simulink model "plant_VV"  (R2023a)
settings: Solver=FixedStepAuto  StartTime=0.0  StopTime=10.0  FixedStep=0.01  RelTol=1e-3
values from neighbouring files (symbols this model uses):
  dt = 0.01    [untitled.m]
  sys = ss(A,B,C,D)    [control_law_design.m]    (also in untitled.m = ss(A,B,C,D, dt))
libraries: simulink_extras x4, shared6dof x1
settings Model: Creator=timme  LastModifiedBy=timme
settings OptimizationCC: BlockReduction=off  DefaultParameterBehavior=Inlined  BufferReuse=off

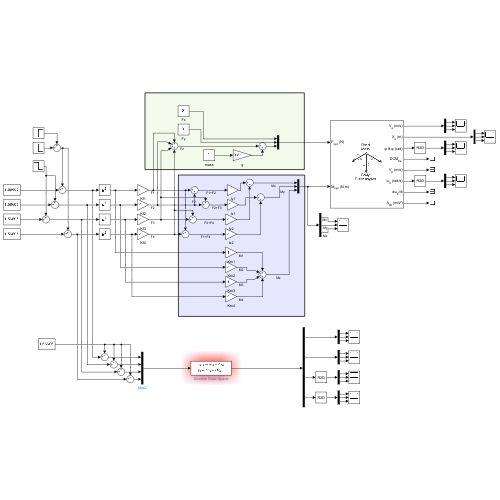
[thumbnail: Simulink's stored preview of the top-level diagram]
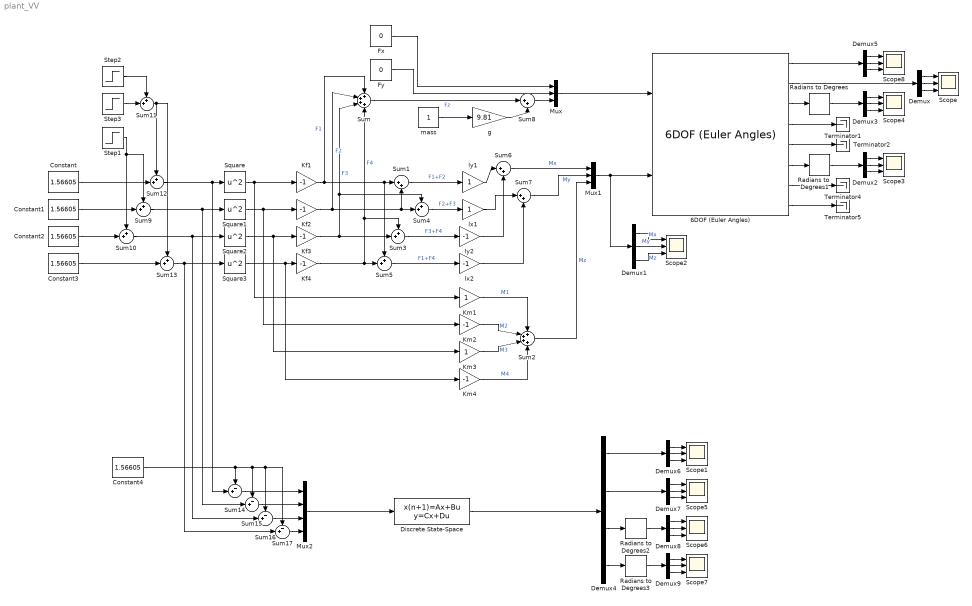
== system plant_VV ==
  6DOF (Euler Angles) : shared6dof/6DOF (Euler Angles)  units=Metric (MKS)  mtype=Fixed  rep=Euler Angles  xme_0=[0 0 0]  Vm_0=[0 0 0]  eul_0=[0 0 0]  pm_0=[0 0 0]  mass_0=1.0  mass_e=0.5  mass_f=2.0  inertia=eye(3)  inertia_e=eye(3)  inertia_f=2*eye(3)  k_quat=1.0  vre_flag=on  abi_flag=off  aMode=0  xme_statename=''  Vm_statename=''  eul_statename=''  quat_statename=''  pm_statename=''  mass_statename=''
  Constant{,1..4} (5 alike) : Constant  Value=1.56605
  Demux{,1..3,5..9} (9 alike) : Demux  Outputs=3
  Demux4 : Demux  Outputs=[3 3 3 3]
  Discrete State-Space : DiscreteStateSpace  A=sys.A  B=sys.B  C=sys.C  D=sys.D  SampleTime=dt
  Fx : Constant  Value=0
  Fy : Constant  Value=0
  Kf{1..4} (4 alike) : Gain  Gain=-1
  Km1 : Gain
  Km2 : Gain  Gain=-1
  Km3 : Gain
  Km4 : Gain  Gain=-1
  Mux : Mux  Inputs=3
  Mux1 : Mux  Inputs=3
  Mux2 : Mux
  Radians to Degrees{,1..3} (4 alike) : simulink_extras/Transformations/Radians to Degrees
  Scope{,1..8} (9 alike) : Scope  NumInputPorts=3
  Square{,1..3} (4 alike) : Math  Operator=square
  Step1 : Step  Time=0.05  Before=0.5  After=0  SampleTime=0
  Step2 : Step  Time=0.05  After=0.5  SampleTime=0
  Step3 : Step  Time=0.1  After=-0.5  SampleTime=0
  Sum : Sum  Inputs=++++
  Sum{1,6..8} (4 alike) : Sum  Inputs=|++
  Sum{3..5,9..13} (8 alike) : Sum  Inputs=++|
  Sum{14..17} (4 alike) : Sum  Inputs=-+|
  Sum2 : Sum  Inputs=++++
  Terminator{1..2,4..5} (4 alike) : Terminator
  g : Gain  Gain=9.81
  lx1 : Gain
  lx2 : Gain  Gain=-1
  ly1 : Gain
  ly2 : Gain  Gain=-1
  mass : Constant
  wires:
  6DOF (Euler Angles)/2 -> Demux/1
  Mux/1 -> 6DOF (Euler Angles)/1
  Constant/1 -> Sum12/2
  Constant1/1 -> Sum9/2
  Square/1 -> Kf1/1, Km1/1
  Square1/1 -> Km2/1, Kf2/1
  Constant2/1 -> Sum10/2
  Square2/1 -> Km3/1, Kf3/1
  Constant3/1 -> Sum13/2
  Square3/1 -> Km4/1, Kf4/1
  Sum/1 -> Sum8/1  "Fz"
  Fx/1 -> Mux/1
  Fy/1 -> Mux/2
  Kf1/1 -> Sum/1, Sum1/1, Sum5/1  "F1"
  Kf2/1 -> Sum/2, Sum4/2, Sum1/2  "F2"
  Kf4/1 -> Sum/4, Sum3/1, Sum5/2  "F4"
  Kf3/1 -> Sum/3, Sum4/1, Sum3/2  "F3"
  Mux1/1 -> Demux1/1, 6DOF (Euler Angles)/2
  Km1/1 -> Sum2/1  "M1"
  Km2/1 -> Sum2/2  "M2"
  Km3/1 -> Sum2/3  "M3"
  Km4/1 -> Sum2/4  "M4"
  Sum2/1 -> Mux1/3  "Mz"
  Sum5/1 -> lx2/1  "F1+F4"
  Sum3/1 -> ly2/1  "F3+F4"
  Sum4/1 -> lx1/1  "F2+F3"
  Sum1/1 -> ly1/1  "F1+F2"
  ly1/1 -> Sum6/1
  ly2/1 -> Sum6/2
  Sum6/1 -> Mux1/1  "Mx"
  Sum7/1 -> Mux1/2  "My"
  lx1/1 -> Sum7/1
  lx2/1 -> Sum7/2
  6DOF (Euler Angles)/4 -> Terminator1/1
  6DOF (Euler Angles)/5 -> Terminator2/1
  6DOF (Euler Angles)/6 -> Radians to Degrees1/1
  6DOF (Euler Angles)/7 -> Terminator4/1
  6DOF (Euler Angles)/8 -> Terminator5/1
  Demux/1 -> Scope/1
  Demux/2 -> Scope/2
  Demux/3 -> Scope/3
  Demux1/2 -> Scope2/2  "My"
  Demux1/1 -> Scope2/1  "Mx"
  Demux1/3 -> Scope2/3  "Mz"
  Sum8/1 -> Mux/3
  mass/1 -> g/1
  g/1 -> Sum8/2
  Step1/1 -> Sum9/1, Sum10/1
  Sum9/1 -> Sum15/2, Square1/1
  Sum10/1 -> Sum16/2, Square2/1
  Demux2/1 -> Scope3/1
  Demux2/3 -> Scope3/3
  Demux2/2 -> Scope3/2
  Demux3/1 -> Scope4/1
  Demux3/3 -> Scope4/3
  6DOF (Euler Angles)/3 -> Radians to Degrees/1
  Demux3/2 -> Scope4/2
  Step3/1 -> Sum11/2
  Step2/1 -> Sum11/1
  Sum11/1 -> Sum13/1, Sum12/1
  Sum12/1 -> Sum14/2, Square/1
  Sum13/1 -> Sum17/2, Square3/1
  Radians to Degrees/1 -> Demux3/1
  Mux2/1 -> Discrete State-Space/1
  Discrete State-Space/1 -> Demux4/1
  6DOF (Euler Angles)/1 -> Demux5/1
  Demux5/3 -> Scope8/3
  Demux5/2 -> Scope8/2
  Demux5/1 -> Scope8/1
  Radians to Degrees1/1 -> Demux2/1
  Sum14/1 -> Mux2/1
  Sum15/1 -> Mux2/2
  Sum16/1 -> Mux2/3
  Sum17/1 -> Mux2/4
  Constant4/1 -> Sum17/1, Sum16/1, Sum15/1, Sum14/1
  Demux4/1 -> Demux6/1
  Demux6/3 -> Scope1/3
  Demux6/2 -> Scope1/2
  Demux6/1 -> Scope1/1
  Demux7/1 -> Scope5/1
  Demux7/2 -> Scope5/2
  Demux7/3 -> Scope5/3
  Demux4/2 -> Demux7/1
  Demux8/1 -> Scope6/1
  Demux8/2 -> Scope6/2
  Demux8/3 -> Scope6/3
  Demux4/3 -> Radians to Degrees2/1
  Radians to Degrees2/1 -> Demux8/1
  Demux4/4 -> Radians to Degrees3/1
  Demux9/3 -> Scope7/3
  Demux9/2 -> Scope7/2
  Demux9/1 -> Scope7/1
  Radians to Degrees3/1 -> Demux9/1
